simulink model "discrete_luenberger"  (R2020b)
settings: Solver=VariableStepAuto  StartTime=0.0  StopTime=10000  RelTol=1e-3
values from neighbouring files (symbols this model uses):
  F_k = k*[1/theta2 -theta3 -theta3]    [script1.m]
undefined symbols (not defined in the file or in its folder): A_foh, A_tustin, A_zoh, B_foh, B_tustin, B_zoh, C_foh, C_tustin, C_zoh, L_foh, L_tustin, L_zoh, Ts
settings Model: Creator=Francesco  LastModifiedBy=Francesco

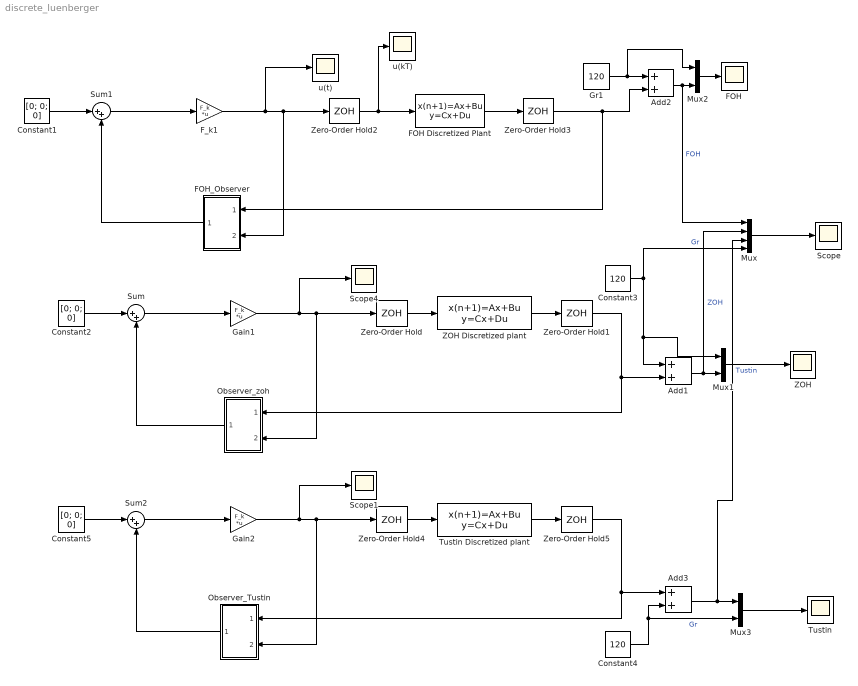
== system discrete_luenberger ==
  Add1 : Sum
  Add2 : Sum
  Add3 : Sum
  Constant1 : Constant  Value=[0; 0; 0]
  Constant2 : Constant  Value=[0; 0; 0]
  Constant3 : Constant  Value=120
  Constant4 : Constant  Value=120
  Constant5 : Constant  Value=[0; 0; 0]
  FOH : Scope
  FOH Discretized Plant : DiscreteStateSpace  A=A_foh  B=B_foh  C=C_foh  D=0  InitialCondition=[130;0;0]  SampleTime=-1
  FOH_Observer : Subsystem
  F_k1 : Gain  Gain=F_k  Multiplication=Matrix(K*u)
  Gain1 : Gain  Gain=F_k  Multiplication=Matrix(K*u)
  Gain2 : Gain  Gain=F_k  Multiplication=Matrix(K*u)
  Gr1 : Constant  Value=120
  Mux : Mux
  Mux1 : Mux  Inputs=2
  Mux2 : Mux  Inputs=2
  Mux3 : Mux  Inputs=2
  Observer_Tustin : Subsystem
  Observer_zoh : Subsystem
  Scope : Scope
  Scope1 : Scope
  Scope4 : Scope
  Sum : Sum  Inputs=|++
  Sum1 : Sum  Inputs=|++
  Sum2 : Sum  Inputs=|++
  Tustin : Scope
  Tustin Discretized plant : DiscreteStateSpace  A=A_tustin  B=B_tustin  C=C_tustin  D=0  InitialCondition=[130;0;0]  SampleTime=-1
  ZOH : Scope
  ZOH Discretized plant : DiscreteStateSpace  A=A_zoh  B=B_zoh  C=C_zoh  D=0  InitialCondition=[130;0;0]  SampleTime=-1
  Zero-Order Hold{,1..5} (6 alike) : ZeroOrderHold  SampleTime=Ts
  u(kT) : Scope
  u(t) : Scope
  wires:
  Mux1/1 -> ZOH/1
  Constant2/1 -> Sum/1
  ZOH Discretized plant/1 -> Zero-Order Hold1/1
  Observer_zoh/1(Out1) -> Sum/2
  Constant3/1 -> Mux/4, Add1/1, Mux1/1  "Gr"
  Sum/1 -> Gain1/1
  Gain1/1 -> Zero-Order Hold/1, Observer_zoh/2(In2), Scope4/1
  Zero-Order Hold/1 -> ZOH Discretized plant/1
  Zero-Order Hold1/1 -> Observer_zoh/1(In1), Add1/2
  Constant1/1 -> Sum1/1
  F_k1/1 -> u(t)/1, Zero-Order Hold2/1, FOH_Observer/2(In2)
  Add2/1 -> Mux/1, Mux2/2  "FOH"
  Gr1/1 -> Add2/1, Mux2/1
  Sum1/1 -> F_k1/1
  FOH_Observer/1(Out1) -> Sum1/2
  FOH Discretized Plant/1 -> Zero-Order Hold3/1
  Mux2/1 -> FOH/1
  Zero-Order Hold2/1 -> FOH Discretized Plant/1, u(kT)/1
  Zero-Order Hold3/1 -> FOH_Observer/1(In1), Add2/2
  Mux/1 -> Scope/1
  Add1/1 -> Mux/2, Mux1/2  "ZOH"
  Tustin Discretized plant/1 -> Zero-Order Hold5/1
  Observer_Tustin/1(Out1) -> Sum2/2
  Zero-Order Hold5/1 -> Observer_Tustin/1(In1), Add3/1
  Zero-Order Hold4/1 -> Tustin Discretized plant/1
  Gain2/1 -> Zero-Order Hold4/1, Observer_Tustin/2(In2), Scope1/1
  Sum2/1 -> Gain2/1
  Constant4/1 -> Mux3/2, Add3/2  "Gr"
  Mux3/1 -> Tustin/1
  Add3/1 -> Mux/3, Mux3/1  "Tustin"
  Constant5/1 -> Sum2/1

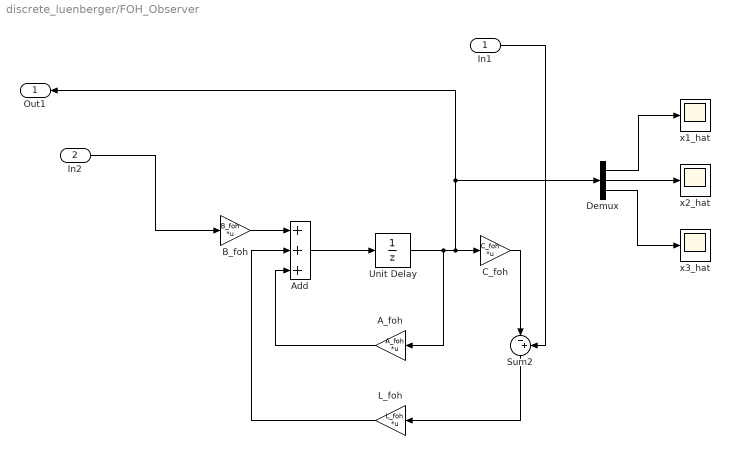
== system discrete_luenberger/FOH_Observer ==
  In1 : Inport
  In2 : Inport  Port=2
  A_foh : Gain  Gain=A_foh  Multiplication=Matrix(K*u)
  Add : Sum  Inputs=+++
  B_foh : Gain  Gain=B_foh  Multiplication=Matrix(K*u)
  C_foh : Gain  Gain=C_foh  Multiplication=Matrix(K*u)
  Demux : Demux  Outputs=3
  L_foh : Gain  Gain=L_foh  Multiplication=Matrix(K*u)
  Sum2 : Sum  Inputs=|-+
  Unit Delay : UnitDelay  SampleTime=-1  HasFrameUpgradeWarning=on
  x1_hat : Scope
  x2_hat : Scope
  x3_hat : Scope
  Out1 : Outport
  wires:
  In1/1 -> Sum2/2
  B_foh/1 -> Add/1
  Sum2/1 -> L_foh/1
  L_foh/1 -> Add/2
  C_foh/1 -> Sum2/1
  A_foh/1 -> Add/3
  Add/1 -> Unit Delay/1
  In2/1 -> B_foh/1
  Demux/1 -> x1_hat/1
  Unit Delay/1 -> A_foh/1, Demux/1, Out1/1, C_foh/1
  Demux/2 -> x2_hat/1
  Demux/3 -> x3_hat/1

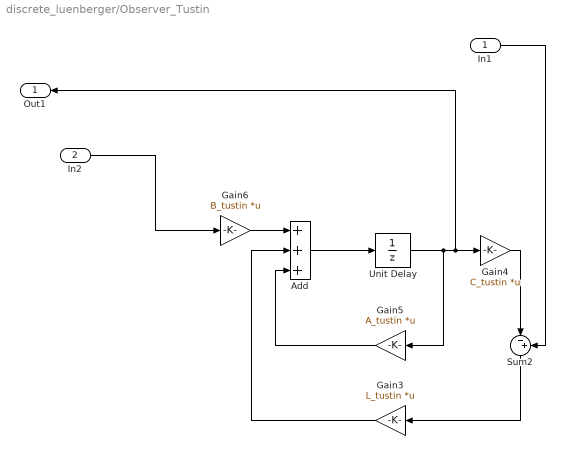
== system discrete_luenberger/Observer_Tustin ==
  In1 : Inport
  In2 : Inport  Port=2
  Add : Sum  Inputs=+++
  Gain3 : Gain  Gain=L_tustin  Multiplication=Matrix(K*u)
  Gain4 : Gain  Gain=C_tustin  Multiplication=Matrix(K*u)
  Gain5 : Gain  Gain=A_tustin  Multiplication=Matrix(K*u)
  Gain6 : Gain  Gain=B_tustin  Multiplication=Matrix(K*u)
  Sum2 : Sum  Inputs=|-+
  Unit Delay : UnitDelay  SampleTime=-1  HasFrameUpgradeWarning=on
  Out1 : Outport
  wires:
  In1/1 -> Sum2/2
  Gain6/1 -> Add/1
  Sum2/1 -> Gain3/1
  Gain3/1 -> Add/2
  Gain4/1 -> Sum2/1
  Gain5/1 -> Add/3
  Add/1 -> Unit Delay/1
  In2/1 -> Gain6/1
  Unit Delay/1 -> Gain5/1, Out1/1, Gain4/1

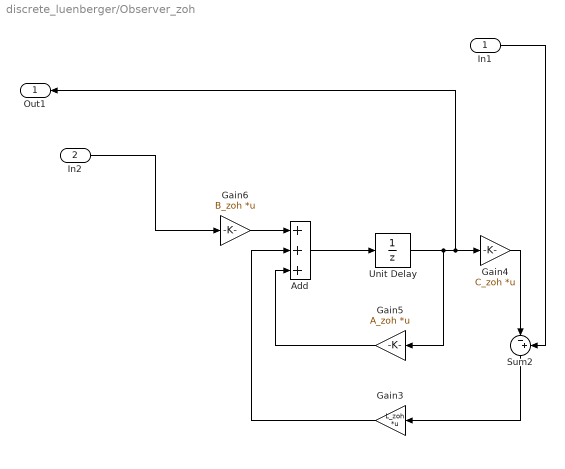
== system discrete_luenberger/Observer_zoh ==
  In1 : Inport
  In2 : Inport  Port=2
  Add : Sum  Inputs=+++
  Gain3 : Gain  Gain=L_zoh  Multiplication=Matrix(K*u)
  Gain4 : Gain  Gain=C_zoh  Multiplication=Matrix(K*u)
  Gain5 : Gain  Gain=A_zoh  Multiplication=Matrix(K*u)
  Gain6 : Gain  Gain=B_zoh  Multiplication=Matrix(K*u)
  Sum2 : Sum  Inputs=|-+
  Unit Delay : UnitDelay  SampleTime=-1  HasFrameUpgradeWarning=on
  Out1 : Outport
  wires:
  In1/1 -> Sum2/2
  Gain6/1 -> Add/1
  Sum2/1 -> Gain3/1
  Gain3/1 -> Add/2
  Gain4/1 -> Sum2/1
  Gain5/1 -> Add/3
  Add/1 -> Unit Delay/1
  In2/1 -> Gain6/1
  Unit Delay/1 -> Gain5/1, Out1/1, Gain4/1
